simulink model "Opt_test"  (R2021b)
settings: Solver=VariableStepAuto  StartTime=0.0  StopTime=0  RelTol=1e-3
settings Model: Creator=The MathWorks, Inc.  LastModifiedBy=rhdej

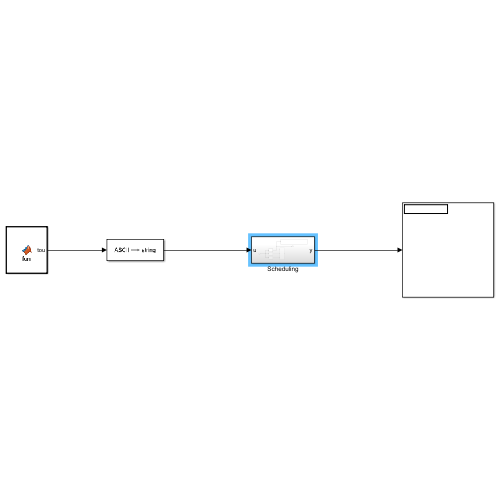
[thumbnail: Simulink's stored preview of the top-level diagram]
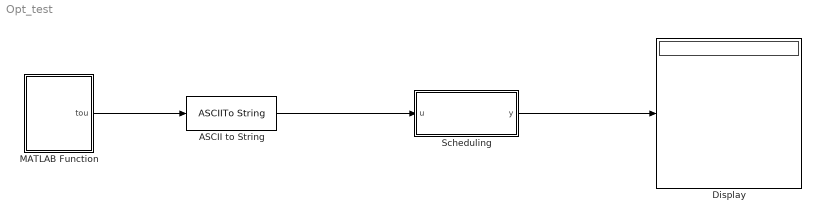
== system Opt_test ==
  ASCII to String : ASCIIToString
  Display : Display
  MATLAB Function : MATLAB Function  TreatAsAtomicUnit=on
  Scheduling : Subsystem
  wires:
  MATLAB Function/1(tou) -> ASCII to String/1
  ASCII to String/1 -> Scheduling/1(u)
  Scheduling/1(y) -> Display/1

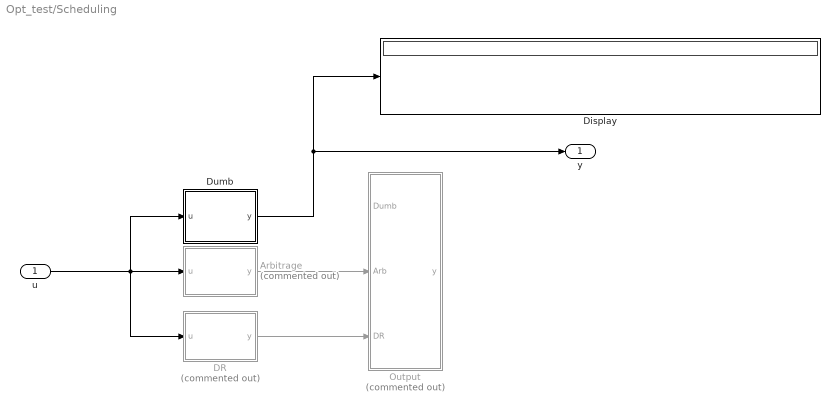
== system Opt_test/Scheduling ==
  u : Inport
  Arbitrage : MATLAB Function  Commented=on  TreatAsAtomicUnit=on
  DR : MATLAB Function  Commented=on  TreatAsAtomicUnit=on
  Display : Display
  Dumb : MATLAB Function  TreatAsAtomicUnit=on
  "Output " : MATLAB Function  Commented=on  TreatAsAtomicUnit=on
  y : Outport
  wires:
  u/1 -> Dumb/1(u), DR/1(u), Arbitrage/1(u)
  Arbitrage/1(y) -> "Output "/2(Arb)
  DR/1(y) -> "Output "/3(DR)
  Dumb/1(y) -> y/1, Display/1

== matlab function Opt_test/Scheduling/Arbitrage ==
  data: u input; y output
function y = Arb(u)
coder.extrinsic("readmatrix")
coder.extrinsic("intlinprog")

input = readmatrix(u);

== matlab function Opt_test/MATLAB Function ==
  data: tou output
%% 데이터 전처리
function tou   = fcn
coder.extrinsic("readtable")
coder.extrinsic("readmatrix")
coder.extrinsic("writematrix")

input_ev = readmatrix("input/evConfig.csv");

writematrix(input_ev,'ev.csv')
filename = 'ev.csv';
tou = uint8(filename);

== matlab function Opt_test/Scheduling/DR ==
  data: u input; y output
function y = DR(u)
coder.extrinsic("readmatrix")
coder.extrinsic("intlinprog")

input = readmatrix(u);

== matlab function Opt_test/Scheduling/Dumb ==
  data: u input; y output
function y = Dumb(u)
coder.extrinsic("readmatrix")
coder.extrinsic("writematrix")

%Day : 1, ID : 2, Cap : 3, Init : 4, Target : 5, Min : 6, Max : 7, In : 8,
%Out : 9, Pmin : 10, Pmax : 11, Mode : 12, Massive option : 13
ev = readmatrix(u);
hour = 48;

size_ev = 0;
size_ev = size(ev,1);
column_ev = 0;
column_ev = size(ev,2);

ev_day0 = zeros(1);
for i = 1:size_ev
    temp = zeros(1);
    temp = ev(i,1);
    idx = temp == 0;
    if idx == 1
        ev_day0 = zeros(i,column_ev);
        ev_day0(1:i,1:column_ev) = ev(1:i,1:column_ev);
    end
end

ev = ev_day0;
size_ev = 0;
size_ev = size(ev,1);
in = zeros(size_ev,1);
out = zeros(size_ev,1);
for i = 1:size_ev
    in(i,1) = ev(i,8);
    out(i,1) = ev(i,9);
end
%%
power = zeros(size_ev,hour);
rate = 5;
for i = 1:size_ev
    ev(i,5) = ev(i,5) * ev(i,3);
    ev(i,4) = ev(i,4) * ev(i,3);
end
Chg_time = zeros(size_ev,1);

for i = 1:size_ev
    Chg_time(i,1) = ceil((ev(i,5) - ev(i,4))/rate);
end

for i = 1:size_ev
    if Chg_time(i,1) >= 0
        if Chg_time(i,1) > 1
            power(i,(in(i,1):in(i,1)+Chg_time(i,1))) = rate;
        elseif Chg_time(i,1) <= 1
            power(i,in(i,1)) = Chg_time(i,1) * rate;
        end
    end
end
writematrix(ev,'test_ev.csv')
writematrix(Chg_time,'test.csv')
writematrix(power,'power.csv')
y = length(power);

end

== matlab function Opt_test/Scheduling/Output  ==
  data: Dumb input; y output; Arb input; DR input
function y = fcn(Dumb, Arb, DR)
coder.extrinsic("readmatrix")
coder.extrinsic("intlinprog")

input = readmatrix(u);
